simulink model "simulink3"  (R2017a)
settings: Solver=VariableStepAuto  StartTime=0.0  StopTime=.5  RelTol=1e-3
libraries: cstblocks x4
settings Model: Creator=Night_Fury  LastModifiedBy=Havoc

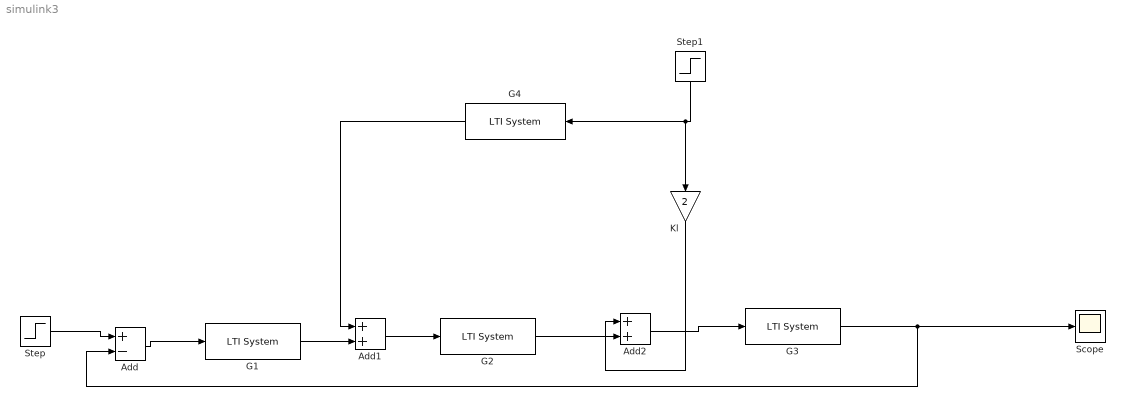
== system simulink3 ==
  Add : Sum  Inputs=+-
  Add1 : Sum
  Add2 : Sum
  G1 : cstblocks/LTI System  sys=tf(1,[1 1])  IC=[]
  G2 : cstblocks/LTI System  sys=tf(1,[1 1 8])  IC=[]
  "G3 " : cstblocks/LTI System  sys=tf(20,[1 1])  IC=[]
  G4 : cstblocks/LTI System  sys=tf(10,[2 1])  IC=[]
  Kl : Gain  Gain=2
  Scope : Scope
  Step : Step  Time=0  SampleTime=0
  Step1 : Step  Time=0  SampleTime=0
  wires:
  Step1/1 -> Kl/1, G4/1
  Step/1 -> Add/1
  "G3 "/1 -> Add/2, Scope/1
  Add/1 -> G1/1
  G1/1 -> Add1/2
  Add1/1 -> G2/1
  G4/1 -> Add1/1
  G2/1 -> Add2/2
  Add2/1 -> "G3 "/1
  Kl/1 -> Add2/1
